simulink model "GyroscopeSimulationID"  (R2021b)
settings: Solver=FixedStepAuto  StartTime=0.0  StopTime=t(end)  FixedStep=Ts  RelTol=1e-3
undefined symbols (not defined in the file): params, x0
libraries: cstblocks x1, vrlib x1
settings Model: Creator=Patrick  LastModifiedBy=tom
settings SolverCC: AlgebraicLoopSolver=TrustRegion
settings DebuggingCC: SFMachineParentedDataDiag=warning

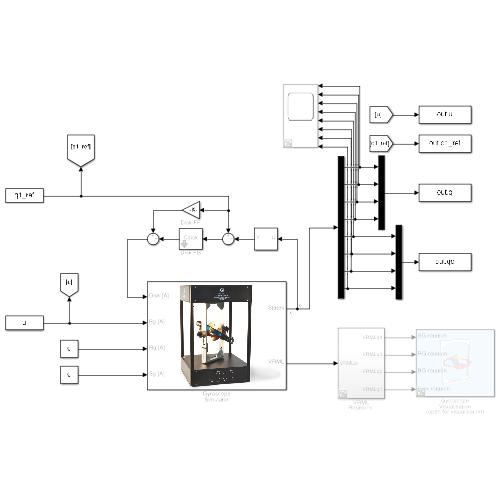
[thumbnail: Simulink's stored preview of the top-level diagram]
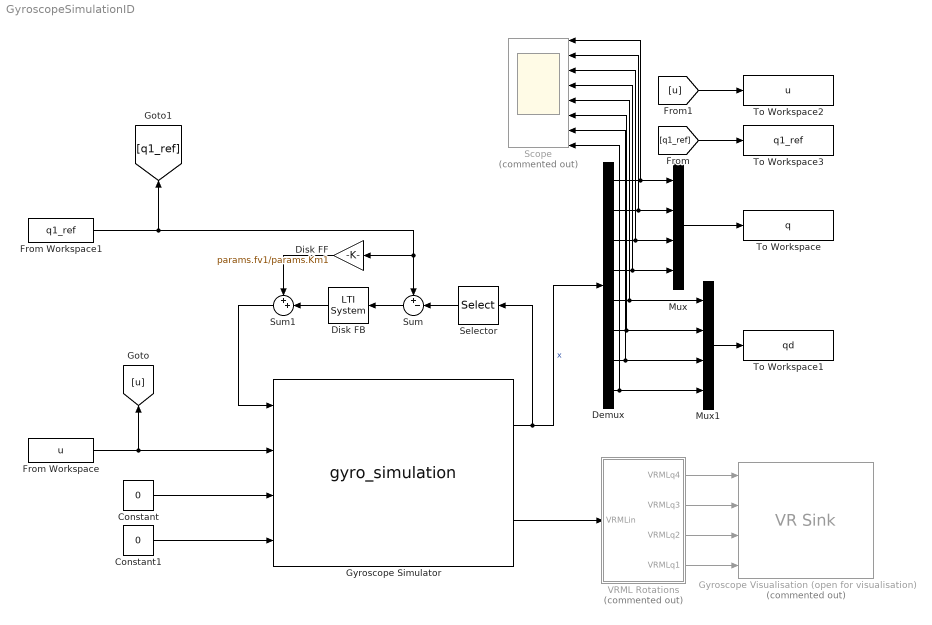
== system GyroscopeSimulationID ==
  Constant : Constant  Value=0
  Constant1 : Constant  Value=0
  Demux : Demux  Outputs=8
  Disk FB : cstblocks/LTI System  sys=Cdisk  IC=[]
  Disk FF : Gain  Gain=params.fv1/params.Km1
  From Workspace : FromWorkspace  VariableName=u
  From Workspace1 : FromWorkspace  VariableName=q1_ref
  Gyroscope Simulator : S-Function  FunctionName=gyro_simulation  Parameters=x0,f,w1l,q2l,q3l,q4l,inertia,Km  SFunctionDeploymentMode=off  EnableBusSupport=off  mask(Gyroscope Simulator){x0=x0, f=[params.fv1;params.fv2;params.fv3;params.fv4], inertia=[params.Ib;params.Ic;params.Id;params.Jb;params.Jc;params.Jd;params.Ka;params.Kb;params.Kc], Km=[params.Km1;params.Km2;params.Km3;params.Km4], w1l=off, q2l=off, q3l=on, q4l=off}
      mask prompts: x0 "Initial conditions (x0):"; f "Viscous friction vector:"; inertia "Inertias:"; Km "Motor constants"; w1l "Disk lock"; q2l "Blue gimbal lock"; q3l "Red gimbal lock"; q4l "Silver gimbal lock"
      mask help:
      | This S-function block simulates the dynamic behavior of the gyroscope setup.
      | Click "Help" for more information.
      mask Help:
      | Outputs are the states of the gyroscope, angular positions and angular velocities, and angles for VRML simulation.
      | The outputs for the states are in the following order:
      | Position disk,
      | Position blue gimbal,
      | Position red gimbal,
      | Position silver gimbal,
      | Velocity disk,
      | Velocity blue gimbal,
      | Velocity red gimbal,
      | Velocity silver gimbal.
      | 
      | Inputs are the torques applied to the following frames:
      | Torque disk,
      | Torque blue gimbal,
      | Torque red gimbal,
      | Torque silver gimbal.
      | 
      | Parameters of the system are the initial conditions "x0" as well as lock options for each frame. The initial conditions should be entered in the same order as the state-outputs are given, seperated by a semicolon.
      | Gyroscope frames can be locked by checking the box for the corresponding frame. In case of locking, the initial conditions can be used to fix a frame under a certain angular position / velocity.
      | 
      | Viscous friction terms can be entered in a [4x1] vector in the order: [disk; blue gimbal; red gimbal; silver gimbal]
      | Inertia parameters can be entered in a [9x1] vector in the order: [Ib;Ic;Id;Jb;Jc;Jd;Ka;Kb;Kc]
      | Motor constants can be entered in a [4x1] vector in the order: [Km1;Km2;Km3;Km4]
      mask DialogControl DescGroupVar Prompt: Gyroscope Simulator
      mask DialogControl DescTextVar Prompt: Simulation block of the Quanser 3 DOF Gyroscope.
      mask DialogControl Gimbal_lock Prompt: Gimbal Lock
      mask Display:
      | disp('dx/dt = f(x,u)\n y = x')
      | image(imread('gyroscope.jpg'))
      | port_label('output',1,'States')
      | port_label('output',2,'VRML')
      | port_label('input',1,'Disk [A]')
      | port_label('input',2,'Bg [A]')
      | port_label('input',3,'Rg [A]')
      | port_label('input',4,'Sg [A]')
  Gyroscope Visualisation (open for visualisation) : vrlib/VR Sink  Commented=on  InstantiateOnLoad=on  SampleTime=-1  ViewEnable=on  RemoteChange=off  RemoteView=off  FieldsWritten=SG.rotation.4.1.1.double#RG.rotation.4.1.1.double#BG.rotation.4.1.1.double#Disk.rotation.4.1.1.double  WorldFileName=World/Gyroscope_Visualisation.wrl  WorldDescription=Gyroscope Visualisation  AutoView=off  VideoDimensions=[]  AllowVariableSize=off
  Mux : Mux
  Mux1 : Mux
  Scope : Scope  Commented=on  NumInputPorts=8
  Selector : Selector  InputPortWidth=8  IndexOptions=Index vector (dialog)  Indices=5  OutputSizes=1
  Sum : Sum  Inputs=+-|
  Sum1 : Sum  Inputs=++|
  To Workspace : ToWorkspace  VariableName=q  SaveFormat=Timeseries  SampleTime=-1
  To Workspace1 : ToWorkspace  VariableName=qd  SaveFormat=Timeseries  SampleTime=-1
  To Workspace2 : ToWorkspace  VariableName=u  SaveFormat=Timeseries  SampleTime=-1
  To Workspace3 : ToWorkspace  VariableName=q1_ref  SaveFormat=Timeseries  SampleTime=-1
  "VRML Rotations " : Subsystem  Commented=on
  wires:
  Gyroscope Simulator/2 -> "VRML Rotations "/1(VRMLin)
  "VRML Rotations "/3(VRMLq2) -> Gyroscope Visualisation (open for visualisation)/3
  "VRML Rotations "/4(VRMLq1) -> Gyroscope Visualisation (open for visualisation)/4
  "VRML Rotations "/1(VRMLq4) -> Gyroscope Visualisation (open for visualisation)/1
  "VRML Rotations "/2(VRMLq3) -> Gyroscope Visualisation (open for visualisation)/2
  Demux/1 -> Scope/1, Mux/1
  Demux/2 -> Scope/2, Mux/2
  Demux/3 -> Scope/3, Mux/3
  Demux/6 -> Mux1/2, Scope/6
  Demux/7 -> Mux1/3, Scope/7
  Demux/8 -> Mux1/4, Scope/8
  Demux/4 -> Scope/4, Mux/4
  Demux/5 -> Mux1/1, Scope/5
  Mux/1 -> To Workspace/1
  Mux1/1 -> To Workspace1/1
  From Workspace/1 -> [u], Gyroscope Simulator/2
  Disk FF/1 -> Sum1/1
  Disk FB/1 -> Sum1/2
  Gyroscope Simulator/1 -> Selector/1, Demux/1  "x"
  Sum/1 -> Disk FB/1
  Selector/1 -> Sum/2
  Sum1/1 -> Gyroscope Simulator/1
  From Workspace1/1 -> [q1_ref], Disk FF/1, Sum/1
  Constant/1 -> Gyroscope Simulator/3
  Constant1/1 -> Gyroscope Simulator/4
  [u] -> To Workspace2/1
  [q1_ref] -> To Workspace3/1

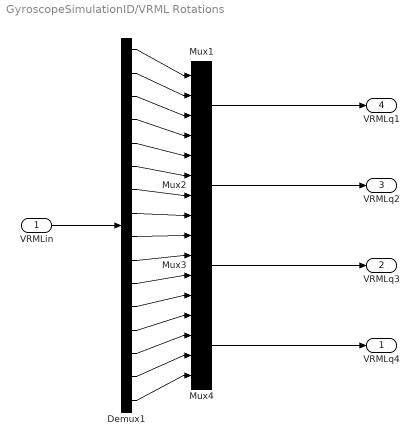
== system GyroscopeSimulationID/VRML Rotations  ==
  VRMLin : Inport
  Demux1 : Demux  Outputs=16
  Mux{1..4} (4 alike) : Mux
  VRMLq4 : Outport
  VRMLq3 : Outport  Port=2
  VRMLq2 : Outport  Port=3
  VRMLq1 : Outport  Port=4
  wires:
  Mux1/1 -> VRMLq1/1
  Demux1/3 -> Mux1/3
  Demux1/8 -> Mux2/4
  Demux1/14 -> Mux4/2
  Demux1/12 -> Mux3/4
  Demux1/11 -> Mux3/3
  Demux1/13 -> Mux4/1
  Demux1/16 -> Mux4/4
  Mux4/1 -> VRMLq4/1
  Demux1/9 -> Mux3/1
  Demux1/7 -> Mux2/3
  Demux1/10 -> Mux3/2
  Demux1/15 -> Mux4/3
  Mux3/1 -> VRMLq3/1
  Mux2/1 -> VRMLq2/1
  Demux1/5 -> Mux2/1
  Demux1/2 -> Mux1/2
  Demux1/4 -> Mux1/4
  Demux1/1 -> Mux1/1
  Demux1/6 -> Mux2/2
  VRMLin/1 -> Demux1/1
